simulink model "VFM_FFL_Inverter_v2"  (R2020b)
settings: Solver=FixedStepAuto  StartTime=0.0  StopTime=6  FixedStep=Ts  RelTol=1e-3
values from neighbouring files (symbols this model uses):
  Cdc = 0.125    [Para.m]    (also in Para_VFM_FFL_Inverter.m = 0.101859163579; Para_VFM_FFL_Inverter_v2.m = 0.101859163579)
  Cf = 0.02    [Para.m]    (also in Para_VFM_FFL_Inverter.m; Para_VFM_FFL_Inverter_v2.m)
  Lc = 0.02    [Para.m]    (also in Para_VFM_FFL_Inverter.m; Para_VFM_FFL_Inverter_v2.m)
  Lf = 0.05    [Para.m]    (also in Para_VFM_FFL_Inverter.m; Para_VFM_FFL_Inverter_v2.m)
  m = 5/100    (= 0.05)    [Para.m]    (also in Para_VFM_FFL_Inverter.m; Para_VFM_FFL_Inverter_v2.m)
  Rdc = w_droop/Wbase*vdc_ref^2    (= 0.625)    [Para_VFM_FFL_Inverter.m]    (also in Para_VFM_FFL_Inverter_v2.m = 0.3125)
  Rline = Xline/5    (= 0.19)    [Para.m]    (also in Para_VFM_FFL_Inverter.m; Para_VFM_FFL_Inverter_v2.m)
  Sbase = 1    [Para.m]    (also in Para_VFM_FFL_Inverter.m; Para_VFM_FFL_Inverter_v2.m)
  Ts = 1/Fs    (= 0.0001)    [Para.m]    (also in Para_VFM_FFL_Inverter.m; Para_VFM_FFL_Inverter_v2.m = 5e-05)
  Vbase = 1    [Para.m]    (also in Para_VFM_FFL_Inverter.m; Para_VFM_FFL_Inverter_v2.m)
  vdc_ref = 2.5    [Para.m]    (also in Para_VFM_FFL_Inverter.m; Para_VFM_FFL_Inverter_v2.m)
  w_droop = 1*2*pi    (= 6.28318530718)    [Para.m]    (also in Para_VFM_FFL_Inverter.m = 31.4159265359; Para_VFM_FFL_Inverter_v2.m = 31.4159265359)
  w_i = 600*2*pi    (= 3769.91118431)    [Para.m]    (also in Para_VFM_FFL_Inverter.m; Para_VFM_FFL_Inverter_v2.m)
  w_v = 300*2*pi    (= 1884.95559215)    [Para.m]    (also in Para_VFM_FFL_Inverter.m; Para_VFM_FFL_Inverter_v2.m)
  Wbase = 2*pi*50    (= 314.159265359)    [Para.m]    (also in Para_VFM_FFL_Inverter.m; Para_VFM_FFL_Inverter_v2.m)
  Xline = 0.95    [Para.m]    (also in Para_VFM_FFL_Inverter.m; Para_VFM_FFL_Inverter_v2.m)
  Zbase = Vbase/Ibase    (= 1)    [Para.m]    (also in Para_VFM_FFL_Inverter.m; Para_VFM_FFL_Inverter_v2.m)
undefined symbols (not defined in the file or in its folder): DiscIntNeverNeededParam, initial
libraries: powerlib x173, SimplusGT x9
(part 4 of 4)

== system VFM_FFL_Inverter_v2/GFM/Current Controller/PI-DT-Estimated d ==
  enable : Inport
  reference : Inport  Port=2
  initial : Inport  Port=3
  actual : Inport  Port=4
  Discrete-Time Integrator : DiscreteIntegrator  gainval=1  ExternalReset=rising  InitialConditionSource=external  InitialCondition=initial  SampleTime=Ts  LimitOutput=on  UpperSaturationLimit=xmax  LowerSaturationLimit=xmin  ICPrevOutput=DiscIntNeverNeededParam  ICPrevScaledInput=DiscIntNeverNeededParam
  Ierror : Sum  Inputs=+-
  Ki : Gain  Gain=Ki  SaturateOnIntegerOverflow=on  OutDataTypeStr=Inherit: Same as input  ParamDataTypeStr=Inherit: Same as input
  Kp : Gain  Gain=Kp  SaturateOnIntegerOverflow=on  OutDataTypeStr=Inherit: Same as input  ParamDataTypeStr=Inherit: Same as input
  Perror : Sum  Inputs=-+
  Product : Product  RndMeth=Zero
  Product1 : Product  RndMeth=Zero
  Saturation : Saturate  UpperLimit=xmax  LowerLimit=xmin
  Sum1 : Sum  SaturateOnIntegerOverflow=on
  Out : Outport
  wires:
  Product1/1 -> Ki/1
  Ierror/1 -> Product1/1
  Product/1 -> Kp/1
  Perror/1 -> Product/1
  reference/1 -> Ierror/1, Perror/2
  actual/1 -> Ierror/2, Perror/1
  initial/1 -> Discrete-Time Integrator/3
  enable/1 -> Product1/2, Product/2, Discrete-Time Integrator/2
  Discrete-Time Integrator/1 -> Sum1/2
  Kp/1 -> Sum1/1
  Ki/1 -> Discrete-Time Integrator/1
  Sum1/1 -> Saturation/1
  Saturation/1 -> Out/1

== system VFM_FFL_Inverter_v2/GFM/Current Controller/PI-DT-Estimated q ==
  actual : Inport
  initial : Inport  Port=2
  reference : Inport  Port=3
  enable : Inport  Port=4
  Discrete-Time Integrator : DiscreteIntegrator  gainval=1  ExternalReset=rising  InitialConditionSource=external  InitialCondition=initial  SampleTime=Ts  LimitOutput=on  UpperSaturationLimit=xmax  LowerSaturationLimit=xmin  ICPrevOutput=DiscIntNeverNeededParam  ICPrevScaledInput=DiscIntNeverNeededParam
  Ierror : Sum  Inputs=+-
  Ki : Gain  Gain=Ki  SaturateOnIntegerOverflow=on  OutDataTypeStr=Inherit: Same as input  ParamDataTypeStr=Inherit: Same as input
  Kp : Gain  Gain=Kp  SaturateOnIntegerOverflow=on  OutDataTypeStr=Inherit: Same as input  ParamDataTypeStr=Inherit: Same as input
  Perror : Sum  Inputs=-+
  Product : Product  RndMeth=Zero
  Product1 : Product  RndMeth=Zero
  Saturation : Saturate  UpperLimit=xmax  LowerLimit=xmin
  Sum1 : Sum  SaturateOnIntegerOverflow=on
  Out : Outport
  wires:
  Product1/1 -> Ki/1
  Ierror/1 -> Product1/1
  Product/1 -> Kp/1
  Perror/1 -> Product/1
  reference/1 -> Ierror/1, Perror/2
  actual/1 -> Perror/1, Ierror/2
  initial/1 -> Discrete-Time Integrator/3
  enable/1 -> Product1/2, Product/2, Discrete-Time Integrator/2
  Discrete-Time Integrator/1 -> Sum1/2
  Kp/1 -> Sum1/1
  Ki/1 -> Discrete-Time Integrator/1
  Sum1/1 -> Saturation/1
  Saturation/1 -> Out/1

== system VFM_FFL_Inverter_v2/GFM/LCL Filter/LL -> LN ==
  note: Transformation from line-to-line voltage to line-to-neutral voltage.
      |
      | Author(s): Yitong Li
  In1 : Inport
  Fcn : Fcn  Expr=u[1]-u[3]
  Fcn1 : Fcn  Expr=u[2]-u[1]
  Fcn2 : Fcn  Expr=u[3]-u[2]
  Gain : Gain  Gain=1/3
  Mux9 : Mux  Inputs=3
  Out1 : Outport
  wires:
  In1/1 -> Gain/1
  Gain/1 -> Fcn/1, Fcn1/1, Fcn2/1
  Mux9/1 -> Out1/1
  Fcn2/1 -> Mux9/3
  Fcn1/1 -> Mux9/2
  Fcn/1 -> Mux9/1

== system VFM_FFL_Inverter_v2/GFM/LCL Filter/LL -> LN1 ==
  note: Transformation from line-to-line voltage to line-to-neutral voltage.
      |
      | Author(s): Yitong Li
  In1 : Inport
  Fcn : Fcn  Expr=u[1]-u[3]
  Fcn1 : Fcn  Expr=u[2]-u[1]
  Fcn2 : Fcn  Expr=u[3]-u[2]
  Gain : Gain  Gain=1/3
  Mux9 : Mux  Inputs=3
  Out1 : Outport
  wires:
  In1/1 -> Gain/1
  Gain/1 -> Fcn/1, Fcn1/1, Fcn2/1
  Mux9/1 -> Out1/1
  Fcn2/1 -> Mux9/3
  Fcn1/1 -> Mux9/2
  Fcn/1 -> Mux9/1

== system VFM_FFL_Inverter_v2/GFM/Voltage Controller/PI-DT-Estimated d ==
  enable : Inport
  reference : Inport  Port=2
  initial : Inport  Port=3
  actual : Inport  Port=4
  Discrete-Time Integrator : DiscreteIntegrator  gainval=1  ExternalReset=rising  InitialConditionSource=external  InitialCondition=initial  SampleTime=Ts  LimitOutput=on  UpperSaturationLimit=xmax  LowerSaturationLimit=xmin  ICPrevOutput=DiscIntNeverNeededParam  ICPrevScaledInput=DiscIntNeverNeededParam
  Ierror : Sum  Inputs=+-
  Ki : Gain  Gain=Ki  SaturateOnIntegerOverflow=on  OutDataTypeStr=Inherit: Same as input  ParamDataTypeStr=Inherit: Same as input
  Kp : Gain  Gain=Kp  SaturateOnIntegerOverflow=on  OutDataTypeStr=Inherit: Same as input  ParamDataTypeStr=Inherit: Same as input
  Perror : Sum  Inputs=-+
  Product : Product  RndMeth=Zero
  Product1 : Product  RndMeth=Zero
  Saturation : Saturate  UpperLimit=xmax  LowerLimit=xmin
  Sum1 : Sum  SaturateOnIntegerOverflow=on
  Out : Outport
  wires:
  Product1/1 -> Ki/1
  Ierror/1 -> Product1/1
  Product/1 -> Kp/1
  Perror/1 -> Product/1
  reference/1 -> Ierror/1, Perror/2
  actual/1 -> Ierror/2, Perror/1
  initial/1 -> Discrete-Time Integrator/3
  enable/1 -> Product1/2, Product/2, Discrete-Time Integrator/2
  Discrete-Time Integrator/1 -> Sum1/2
  Kp/1 -> Sum1/1
  Ki/1 -> Discrete-Time Integrator/1
  Sum1/1 -> Saturation/1
  Saturation/1 -> Out/1

== system VFM_FFL_Inverter_v2/GFM/Voltage Controller/PI-DT-Estimated q ==
  actual : Inport
  initial : Inport  Port=2
  reference : Inport  Port=3
  enable : Inport  Port=4
  Discrete-Time Integrator : DiscreteIntegrator  gainval=1  ExternalReset=rising  InitialConditionSource=external  InitialCondition=initial  SampleTime=Ts  LimitOutput=on  UpperSaturationLimit=xmax  LowerSaturationLimit=xmin  ICPrevOutput=DiscIntNeverNeededParam  ICPrevScaledInput=DiscIntNeverNeededParam
  Ierror : Sum  Inputs=+-
  Ki : Gain  Gain=Ki  SaturateOnIntegerOverflow=on  OutDataTypeStr=Inherit: Same as input  ParamDataTypeStr=Inherit: Same as input
  Kp : Gain  Gain=Kp  SaturateOnIntegerOverflow=on  OutDataTypeStr=Inherit: Same as input  ParamDataTypeStr=Inherit: Same as input
  Perror : Sum  Inputs=-+
  Product : Product  RndMeth=Zero
  Product1 : Product  RndMeth=Zero
  Saturation : Saturate  UpperLimit=xmax  LowerLimit=xmin
  Sum1 : Sum  SaturateOnIntegerOverflow=on
  Out : Outport
  wires:
  Product1/1 -> Ki/1
  Ierror/1 -> Product1/1
  Product/1 -> Kp/1
  Perror/1 -> Product/1
  reference/1 -> Ierror/1, Perror/2
  actual/1 -> Perror/1, Ierror/2
  initial/1 -> Discrete-Time Integrator/3
  enable/1 -> Product1/2, Product/2, Discrete-Time Integrator/2
  Discrete-Time Integrator/1 -> Sum1/2
  Kp/1 -> Sum1/1
  Ki/1 -> Discrete-Time Integrator/1
  Sum1/1 -> Saturation/1
  Saturation/1 -> Out/1

== system VFM_FFL_Inverter_v2/PI GFM/Current Controller/PI-DT-Estimated d ==
  enable : Inport
  reference : Inport  Port=2
  initial : Inport  Port=3
  actual : Inport  Port=4
  Discrete-Time Integrator : DiscreteIntegrator  gainval=1  ExternalReset=rising  InitialConditionSource=external  InitialCondition=initial  SampleTime=Ts  LimitOutput=on  UpperSaturationLimit=xmax  LowerSaturationLimit=xmin  ICPrevOutput=DiscIntNeverNeededParam  ICPrevScaledInput=DiscIntNeverNeededParam
  Ierror : Sum  Inputs=+-
  Ki : Gain  Gain=Ki  SaturateOnIntegerOverflow=on  OutDataTypeStr=Inherit: Same as input  ParamDataTypeStr=Inherit: Same as input
  Kp : Gain  Gain=Kp  SaturateOnIntegerOverflow=on  OutDataTypeStr=Inherit: Same as input  ParamDataTypeStr=Inherit: Same as input
  Perror : Sum  Inputs=-+
  Product : Product  RndMeth=Zero
  Product1 : Product  RndMeth=Zero
  Saturation : Saturate  UpperLimit=xmax  LowerLimit=xmin
  Sum1 : Sum  SaturateOnIntegerOverflow=on
  Out : Outport
  wires:
  Product1/1 -> Ki/1
  Ierror/1 -> Product1/1
  Product/1 -> Kp/1
  Perror/1 -> Product/1
  reference/1 -> Ierror/1, Perror/2
  actual/1 -> Ierror/2, Perror/1
  initial/1 -> Discrete-Time Integrator/3
  enable/1 -> Product1/2, Product/2, Discrete-Time Integrator/2
  Discrete-Time Integrator/1 -> Sum1/2
  Kp/1 -> Sum1/1
  Ki/1 -> Discrete-Time Integrator/1
  Sum1/1 -> Saturation/1
  Saturation/1 -> Out/1

== system VFM_FFL_Inverter_v2/PI GFM/Current Controller/PI-DT-Estimated q ==
  actual : Inport
  initial : Inport  Port=2
  reference : Inport  Port=3
  enable : Inport  Port=4
  Discrete-Time Integrator : DiscreteIntegrator  gainval=1  ExternalReset=rising  InitialConditionSource=external  InitialCondition=initial  SampleTime=Ts  LimitOutput=on  UpperSaturationLimit=xmax  LowerSaturationLimit=xmin  ICPrevOutput=DiscIntNeverNeededParam  ICPrevScaledInput=DiscIntNeverNeededParam
  Ierror : Sum  Inputs=+-
  Ki : Gain  Gain=Ki  SaturateOnIntegerOverflow=on  OutDataTypeStr=Inherit: Same as input  ParamDataTypeStr=Inherit: Same as input
  Kp : Gain  Gain=Kp  SaturateOnIntegerOverflow=on  OutDataTypeStr=Inherit: Same as input  ParamDataTypeStr=Inherit: Same as input
  Perror : Sum  Inputs=-+
  Product : Product  RndMeth=Zero
  Product1 : Product  RndMeth=Zero
  Saturation : Saturate  UpperLimit=xmax  LowerLimit=xmin
  Sum1 : Sum  SaturateOnIntegerOverflow=on
  Out : Outport
  wires:
  Product1/1 -> Ki/1
  Ierror/1 -> Product1/1
  Product/1 -> Kp/1
  Perror/1 -> Product/1
  reference/1 -> Ierror/1, Perror/2
  actual/1 -> Perror/1, Ierror/2
  initial/1 -> Discrete-Time Integrator/3
  enable/1 -> Product1/2, Product/2, Discrete-Time Integrator/2
  Discrete-Time Integrator/1 -> Sum1/2
  Kp/1 -> Sum1/1
  Ki/1 -> Discrete-Time Integrator/1
  Sum1/1 -> Saturation/1
  Saturation/1 -> Out/1

== system VFM_FFL_Inverter_v2/PI GFM/LCL Filter/LL -> LN ==
  note: Transformation from line-to-line voltage to line-to-neutral voltage.
      |
      | Author(s): Yitong Li
  In1 : Inport
  Fcn : Fcn  Expr=u[1]-u[3]
  Fcn1 : Fcn  Expr=u[2]-u[1]
  Fcn2 : Fcn  Expr=u[3]-u[2]
  Gain : Gain  Gain=1/3
  Mux9 : Mux  Inputs=3
  Out1 : Outport
  wires:
  In1/1 -> Gain/1
  Gain/1 -> Fcn/1, Fcn1/1, Fcn2/1
  Mux9/1 -> Out1/1
  Fcn2/1 -> Mux9/3
  Fcn1/1 -> Mux9/2
  Fcn/1 -> Mux9/1

== system VFM_FFL_Inverter_v2/PI GFM/LCL Filter/LL -> LN1 ==
  note: Transformation from line-to-line voltage to line-to-neutral voltage.
      |
      | Author(s): Yitong Li
  In1 : Inport
  Fcn : Fcn  Expr=u[1]-u[3]
  Fcn1 : Fcn  Expr=u[2]-u[1]
  Fcn2 : Fcn  Expr=u[3]-u[2]
  Gain : Gain  Gain=1/3
  Mux9 : Mux  Inputs=3
  Out1 : Outport
  wires:
  In1/1 -> Gain/1
  Gain/1 -> Fcn/1, Fcn1/1, Fcn2/1
  Mux9/1 -> Out1/1
  Fcn2/1 -> Mux9/3
  Fcn1/1 -> Mux9/2
  Fcn/1 -> Mux9/1

== system VFM_FFL_Inverter_v2/PI GFM/PLL (iabc -> id)/Discrete PI ==
  note: Digital PI controller
      |
      | Author(s): Yitong Li
  enable : Inport
  reference : Inport  Port=2
  initial : Inport  Port=3
  actual : Inport  Port=4
  Discrete-Time Integrator : DiscreteIntegrator  gainval=1  ExternalReset=rising  InitialConditionSource=external  InitialCondition=initial  SampleTime=Ts  LimitOutput=on  UpperSaturationLimit=xmax  LowerSaturationLimit=xmin  ICPrevOutput=DiscIntNeverNeededParam  ICPrevScaledInput=DiscIntNeverNeededParam
  Ierror : Sum  Inputs=+-
  Ki : Gain  Gain=Ki  SaturateOnIntegerOverflow=on  OutDataTypeStr=Inherit: Same as input  ParamDataTypeStr=Inherit: Same as input
  Kp : Gain  Gain=Kp  SaturateOnIntegerOverflow=on  OutDataTypeStr=Inherit: Same as input  ParamDataTypeStr=Inherit: Same as input
  Perror : Sum  Inputs=-+
  Product : Product  RndMeth=Zero
  Product1 : Product  RndMeth=Zero
  Saturation : Saturate  UpperLimit=xmax  LowerLimit=xmin
  Sum1 : Sum  SaturateOnIntegerOverflow=on
  Out : Outport
  wires:
  Product1/1 -> Ki/1
  Ierror/1 -> Product1/1
  Product/1 -> Kp/1
  Perror/1 -> Product/1
  actual/1 -> Perror/1, Ierror/2
  reference/1 -> Ierror/1, Perror/2
  initial/1 -> Discrete-Time Integrator/3
  enable/1 -> Product1/2, Product/2, Discrete-Time Integrator/2
  Discrete-Time Integrator/1 -> Sum1/2
  Kp/1 -> Sum1/1
  Ki/1 -> Discrete-Time Integrator/1
  Sum1/1 -> Saturation/1
  Saturation/1 -> Out/1

== system VFM_FFL_Inverter_v2/PI GFM/PLL (iabc -> id)/abc -> dq (Power-Invariant) ==
  note: Frame transformation from abc to dq.
      |
      | Author(s): Yitong Li
      |
      | Notes:
      |
      | The transformation is power-invariant.
      |
      | theta is the angle that d axis leads a axis.
      |
      | q axis leads d axis by 90 degrees.
  abc : Inport
  theta : Inport  Port=2
  ->d : Fcn  Expr=cos(u(4))*u(1) + cos(u(4)-2/3*pi)*u(2) + cos(u(4)-4/3*pi)*u(3)
  ->q : Fcn  Expr=-sin(u(4))*u(1) - sin(u(4)-2/3*pi)*u(2) - sin(u(4)-4/3*pi)*u(3)
  Gain : Gain  Gain=sqrt(2/3)
  Mux5 : Mux  Inputs=2
  Mux6 : Mux  Inputs=2
  dq : Outport
  wires:
  abc/1 -> Gain/1
  ->d/1 -> Mux6/1
  Gain/1 -> Mux5/1
  theta/1 -> Mux5/2
  ->q/1 -> Mux6/2
  Mux6/1 -> dq/1
  Mux5/1 -> ->d/1, ->q/1

== system VFM_FFL_Inverter_v2/PI GFM/Voltage Controller/PI-DT-Estimated d ==
  enable : Inport
  reference : Inport  Port=2
  initial : Inport  Port=3
  actual : Inport  Port=4
  Discrete-Time Integrator : DiscreteIntegrator  gainval=1  ExternalReset=rising  InitialConditionSource=external  InitialCondition=initial  SampleTime=Ts  LimitOutput=on  UpperSaturationLimit=xmax  LowerSaturationLimit=xmin  ICPrevOutput=DiscIntNeverNeededParam  ICPrevScaledInput=DiscIntNeverNeededParam
  Ierror : Sum  Inputs=+-
  Ki : Gain  Gain=Ki  SaturateOnIntegerOverflow=on  OutDataTypeStr=Inherit: Same as input  ParamDataTypeStr=Inherit: Same as input
  Kp : Gain  Gain=Kp  SaturateOnIntegerOverflow=on  OutDataTypeStr=Inherit: Same as input  ParamDataTypeStr=Inherit: Same as input
  Perror : Sum  Inputs=-+
  Product : Product  RndMeth=Zero
  Product1 : Product  RndMeth=Zero
  Saturation : Saturate  UpperLimit=xmax  LowerLimit=xmin
  Sum1 : Sum  SaturateOnIntegerOverflow=on
  Out : Outport
  wires:
  Product1/1 -> Ki/1
  Ierror/1 -> Product1/1
  Product/1 -> Kp/1
  Perror/1 -> Product/1
  reference/1 -> Ierror/1, Perror/2
  actual/1 -> Ierror/2, Perror/1
  initial/1 -> Discrete-Time Integrator/3
  enable/1 -> Product1/2, Product/2, Discrete-Time Integrator/2
  Discrete-Time Integrator/1 -> Sum1/2
  Kp/1 -> Sum1/1
  Ki/1 -> Discrete-Time Integrator/1
  Sum1/1 -> Saturation/1
  Saturation/1 -> Out/1

== system VFM_FFL_Inverter_v2/PI GFM/Voltage Controller/PI-DT-Estimated q ==
  actual : Inport
  initial : Inport  Port=2
  reference : Inport  Port=3
  enable : Inport  Port=4
  Discrete-Time Integrator : DiscreteIntegrator  gainval=1  ExternalReset=rising  InitialConditionSource=external  InitialCondition=initial  SampleTime=Ts  LimitOutput=on  UpperSaturationLimit=xmax  LowerSaturationLimit=xmin  ICPrevOutput=DiscIntNeverNeededParam  ICPrevScaledInput=DiscIntNeverNeededParam
  Ierror : Sum  Inputs=+-
  Ki : Gain  Gain=Ki  SaturateOnIntegerOverflow=on  OutDataTypeStr=Inherit: Same as input  ParamDataTypeStr=Inherit: Same as input
  Kp : Gain  Gain=Kp  SaturateOnIntegerOverflow=on  OutDataTypeStr=Inherit: Same as input  ParamDataTypeStr=Inherit: Same as input
  Perror : Sum  Inputs=-+
  Product : Product  RndMeth=Zero
  Product1 : Product  RndMeth=Zero
  Saturation : Saturate  UpperLimit=xmax  LowerLimit=xmin
  Sum1 : Sum  SaturateOnIntegerOverflow=on
  Out : Outport
  wires:
  Product1/1 -> Ki/1
  Ierror/1 -> Product1/1
  Product/1 -> Kp/1
  Perror/1 -> Product/1
  reference/1 -> Ierror/1, Perror/2
  actual/1 -> Perror/1, Ierror/2
  initial/1 -> Discrete-Time Integrator/3
  enable/1 -> Product1/2, Product/2, Discrete-Time Integrator/2
  Discrete-Time Integrator/1 -> Sum1/2
  Kp/1 -> Sum1/1
  Ki/1 -> Discrete-Time Integrator/1
  Sum1/1 -> Saturation/1
  Saturation/1 -> Out/1

== system VFM_FFL_Inverter_v2/VFM-FFL/Current Controller/PI-DT-Estimated d ==
  enable : Inport
  reference : Inport  Port=2
  initial : Inport  Port=3
  actual : Inport  Port=4
  Discrete-Time Integrator : DiscreteIntegrator  gainval=1  ExternalReset=rising  InitialConditionSource=external  InitialCondition=initial  SampleTime=Ts  LimitOutput=on  UpperSaturationLimit=xmax  LowerSaturationLimit=xmin  ICPrevOutput=DiscIntNeverNeededParam  ICPrevScaledInput=DiscIntNeverNeededParam
  Ierror : Sum  Inputs=+-
  Ki : Gain  Gain=Ki  SaturateOnIntegerOverflow=on  OutDataTypeStr=Inherit: Same as input  ParamDataTypeStr=Inherit: Same as input
  Kp : Gain  Gain=Kp  SaturateOnIntegerOverflow=on  OutDataTypeStr=Inherit: Same as input  ParamDataTypeStr=Inherit: Same as input
  Perror : Sum  Inputs=-+
  Product : Product  RndMeth=Zero
  Product1 : Product  RndMeth=Zero
  Saturation : Saturate  UpperLimit=xmax  LowerLimit=xmin
  Sum1 : Sum  SaturateOnIntegerOverflow=on
  Out : Outport
  wires:
  Product1/1 -> Ki/1
  Ierror/1 -> Product1/1
  Product/1 -> Kp/1
  Perror/1 -> Product/1
  reference/1 -> Ierror/1, Perror/2
  actual/1 -> Ierror/2, Perror/1
  initial/1 -> Discrete-Time Integrator/3
  enable/1 -> Product1/2, Product/2, Discrete-Time Integrator/2
  Discrete-Time Integrator/1 -> Sum1/2
  Kp/1 -> Sum1/1
  Ki/1 -> Discrete-Time Integrator/1
  Sum1/1 -> Saturation/1
  Saturation/1 -> Out/1

== system VFM_FFL_Inverter_v2/VFM-FFL/Current Controller/PI-DT-Estimated q ==
  actual : Inport
  initial : Inport  Port=2
  reference : Inport  Port=3
  enable : Inport  Port=4
  Discrete-Time Integrator : DiscreteIntegrator  gainval=1  ExternalReset=rising  InitialConditionSource=external  InitialCondition=initial  SampleTime=Ts  LimitOutput=on  UpperSaturationLimit=xmax  LowerSaturationLimit=xmin  ICPrevOutput=DiscIntNeverNeededParam  ICPrevScaledInput=DiscIntNeverNeededParam
  Ierror : Sum  Inputs=+-
  Ki : Gain  Gain=Ki  SaturateOnIntegerOverflow=on  OutDataTypeStr=Inherit: Same as input  ParamDataTypeStr=Inherit: Same as input
  Kp : Gain  Gain=Kp  SaturateOnIntegerOverflow=on  OutDataTypeStr=Inherit: Same as input  ParamDataTypeStr=Inherit: Same as input
  Perror : Sum  Inputs=-+
  Product : Product  RndMeth=Zero
  Product1 : Product  RndMeth=Zero
  Saturation : Saturate  UpperLimit=xmax  LowerLimit=xmin
  Sum1 : Sum  SaturateOnIntegerOverflow=on
  Out : Outport
  wires:
  Product1/1 -> Ki/1
  Ierror/1 -> Product1/1
  Product/1 -> Kp/1
  Perror/1 -> Product/1
  reference/1 -> Ierror/1, Perror/2
  actual/1 -> Perror/1, Ierror/2
  initial/1 -> Discrete-Time Integrator/3
  enable/1 -> Product1/2, Product/2, Discrete-Time Integrator/2
  Discrete-Time Integrator/1 -> Sum1/2
  Kp/1 -> Sum1/1
  Ki/1 -> Discrete-Time Integrator/1
  Sum1/1 -> Saturation/1
  Saturation/1 -> Out/1

== system VFM_FFL_Inverter_v2/VFM-FFL/LCL Filter/LL -> LN ==
  note: Transformation from line-to-line voltage to line-to-neutral voltage.
      |
      | Author(s): Yitong Li
  In1 : Inport
  Fcn : Fcn  Expr=u[1]-u[3]
  Fcn1 : Fcn  Expr=u[2]-u[1]
  Fcn2 : Fcn  Expr=u[3]-u[2]
  Gain : Gain  Gain=1/3
  Mux9 : Mux  Inputs=3
  Out1 : Outport
  wires:
  In1/1 -> Gain/1
  Gain/1 -> Fcn/1, Fcn1/1, Fcn2/1
  Mux9/1 -> Out1/1
  Fcn2/1 -> Mux9/3
  Fcn1/1 -> Mux9/2
  Fcn/1 -> Mux9/1

== system VFM_FFL_Inverter_v2/VFM-FFL/LCL Filter/LL -> LN1 ==
  note: Transformation from line-to-line voltage to line-to-neutral voltage.
      |
      | Author(s): Yitong Li
  In1 : Inport
  Fcn : Fcn  Expr=u[1]-u[3]
  Fcn1 : Fcn  Expr=u[2]-u[1]
  Fcn2 : Fcn  Expr=u[3]-u[2]
  Gain : Gain  Gain=1/3
  Mux9 : Mux  Inputs=3
  Out1 : Outport
  wires:
  In1/1 -> Gain/1
  Gain/1 -> Fcn/1, Fcn1/1, Fcn2/1
  Mux9/1 -> Out1/1
  Fcn2/1 -> Mux9/3
  Fcn1/1 -> Mux9/2
  Fcn/1 -> Mux9/1

== system VFM_FFL_Inverter_v2/VFM-FFL/Voltage Controller/PI-DT-Estimated d ==
  enable : Inport
  reference : Inport  Port=2
  initial : Inport  Port=3
  actual : Inport  Port=4
  Discrete-Time Integrator : DiscreteIntegrator  gainval=1  ExternalReset=rising  InitialConditionSource=external  InitialCondition=initial  SampleTime=Ts  LimitOutput=on  UpperSaturationLimit=xmax  LowerSaturationLimit=xmin  ICPrevOutput=DiscIntNeverNeededParam  ICPrevScaledInput=DiscIntNeverNeededParam
  Ierror : Sum  Inputs=+-
  Ki : Gain  Gain=Ki  SaturateOnIntegerOverflow=on  OutDataTypeStr=Inherit: Same as input  ParamDataTypeStr=Inherit: Same as input
  Kp : Gain  Gain=Kp  SaturateOnIntegerOverflow=on  OutDataTypeStr=Inherit: Same as input  ParamDataTypeStr=Inherit: Same as input
  Perror : Sum  Inputs=-+
  Product : Product  RndMeth=Zero
  Product1 : Product  RndMeth=Zero
  Saturation : Saturate  UpperLimit=xmax  LowerLimit=xmin
  Sum1 : Sum  SaturateOnIntegerOverflow=on
  Out : Outport
  wires:
  Product1/1 -> Ki/1
  Ierror/1 -> Product1/1
  Product/1 -> Kp/1
  Perror/1 -> Product/1
  reference/1 -> Ierror/1, Perror/2
  actual/1 -> Ierror/2, Perror/1
  initial/1 -> Discrete-Time Integrator/3
  enable/1 -> Product1/2, Product/2, Discrete-Time Integrator/2
  Discrete-Time Integrator/1 -> Sum1/2
  Kp/1 -> Sum1/1
  Ki/1 -> Discrete-Time Integrator/1
  Sum1/1 -> Saturation/1
  Saturation/1 -> Out/1

== system VFM_FFL_Inverter_v2/VFM-FFL/Voltage Controller/PI-DT-Estimated q ==
  actual : Inport
  initial : Inport  Port=2
  reference : Inport  Port=3
  enable : Inport  Port=4
  Discrete-Time Integrator : DiscreteIntegrator  gainval=1  ExternalReset=rising  InitialConditionSource=external  InitialCondition=initial  SampleTime=Ts  LimitOutput=on  UpperSaturationLimit=xmax  LowerSaturationLimit=xmin  ICPrevOutput=DiscIntNeverNeededParam  ICPrevScaledInput=DiscIntNeverNeededParam
  Ierror : Sum  Inputs=+-
  Ki : Gain  Gain=Ki  SaturateOnIntegerOverflow=on  OutDataTypeStr=Inherit: Same as input  ParamDataTypeStr=Inherit: Same as input
  Kp : Gain  Gain=Kp  SaturateOnIntegerOverflow=on  OutDataTypeStr=Inherit: Same as input  ParamDataTypeStr=Inherit: Same as input
  Perror : Sum  Inputs=-+
  Product : Product  RndMeth=Zero
  Product1 : Product  RndMeth=Zero
  Saturation : Saturate  UpperLimit=xmax  LowerLimit=xmin
  Sum1 : Sum  SaturateOnIntegerOverflow=on
  Out : Outport
  wires:
  Product1/1 -> Ki/1
  Ierror/1 -> Product1/1
  Product/1 -> Kp/1
  Perror/1 -> Product/1
  reference/1 -> Ierror/1, Perror/2
  actual/1 -> Perror/1, Ierror/2
  initial/1 -> Discrete-Time Integrator/3
  enable/1 -> Product1/2, Product/2, Discrete-Time Integrator/2
  Discrete-Time Integrator/1 -> Sum1/2
  Kp/1 -> Sum1/1
  Ki/1 -> Discrete-Time Integrator/1
  Sum1/1 -> Saturation/1
  Saturation/1 -> Out/1
